simulink model "Bands7"  (R2018a)
settings: Solver=VariableStepAuto  StartTime=0.0  StopTime=0.01  RelTol=1e-3
undefined symbols (not defined in the file): fdesignblkfcn, G1, G2, G3, G4, G5, G6, G7, gcbh, get, T
libraries: dspsrcs4 x1, dspxfrm3 x1, dspobslib x1
(part 1 of 2)
settings Model: Creator=Daniel  LastModifiedBy=Daniel

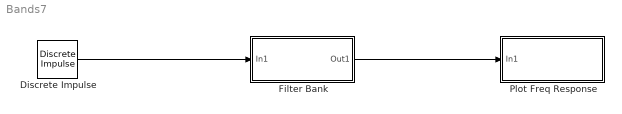
== system Bands7 ==
  Discrete Impulse : dspsrcs4/Discrete  Impulse  Delay=0  SampleTime=T  FrameSample=128  OutputFrames=off  dataType=double  isSigned=on  wordLen=16  udDataType=sfix(16)  fracBitsMode=Best precision  numFracBits=15  OutDataTypeStr=double  LastOutDataTypeStr=double
  "Filter Bank " : Subsystem
  Plot Freq Response : Subsystem
  wires:
  Discrete Impulse/1 -> "Filter Bank "/1(In1)
  "Filter Bank "/1(Out1) -> Plot Freq Response/1(In1)

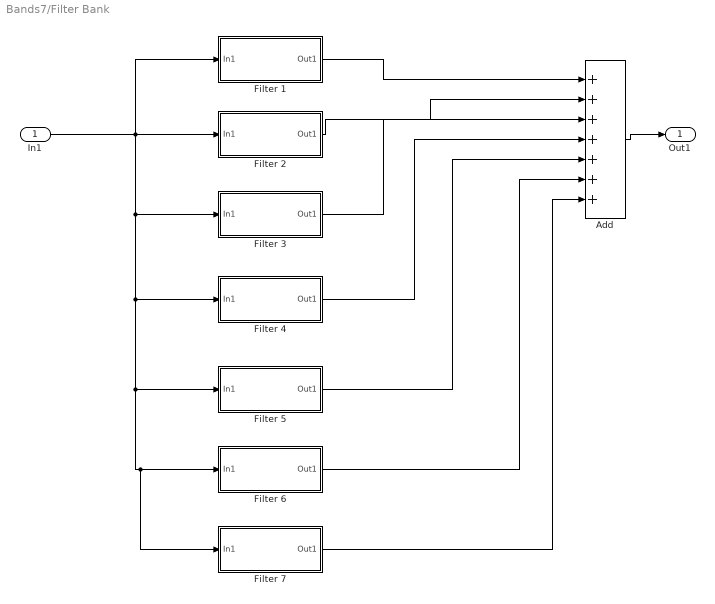
== system Bands7/Filter Bank  ==
  In1 : Inport
  Add : Sum  Inputs=+++++++
  Filter 1 : Subsystem
  Filter 2 : Subsystem
  Filter 3 : Subsystem
  Filter 4 : Subsystem
  Filter 5 : Subsystem
  Filter 6 : Subsystem
  Filter 7 : Subsystem
  Out1 : Outport
  wires:
  In1/1 -> Filter 3/1(In1), Filter 7/1(In1), Filter 6/1(In1), Filter 5/1(In1), Filter 4/1(In1), Filter 1/1(In1), Filter 2/1(In1)
  Add/1 -> Out1/1
  Filter 1/1(Out1) -> Add/1
  Filter 2/1(Out1) -> Add/2
  Filter 3/1(Out1) -> Add/3
  Filter 4/1(Out1) -> Add/4
  Filter 5/1(Out1) -> Add/5
  Filter 6/1(Out1) -> Add/6
  Filter 7/1(Out1) -> Add/7

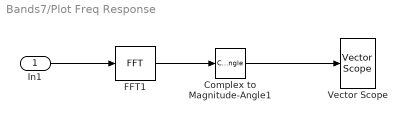
== system Bands7/Plot Freq Response ==
  In1 : Inport
  Complex to Magnitude-Angle1 : ComplexToMagnitudeAngle  Output=Magnitude
  FFT1 : dspxfrm3/FFT  FFTImplementation=Auto  CompMethod=Table lookup  TableOpt=NEW  TableOptActive=Speed  BitRevOrder=off  Normalize=off  InheritFFTLength=on  FFTLength=64  WrapInput=on  roundingMode=Floor  overflowMode=off  firstCoeffDataTypeStr=Inherit: Same word length as input  firstCoeffLastDataTypeStr=Inherit: Same word length as input  outputMin=[]  outputMax=[]
  Vector Scope : dspobslib/Vector Scope  ScopeProperties=off  Domain=Frequency  HorizSpan=1  DisplayProperties=off  AxisGrid=on  Memory=off  FrameNumber=off  AxisLegend=off  AxisZoom=off  OpenScopeAtSimStart=on  OpenScopeImmediately=off  FigPos=get(0,'defaultfigureposition')  AxisProperties=on  XUnits=Hertz  XRange=[0...Fs/2]  InheritXIncr=on  XIncr=1  XLabel=Samples  XLimit=Auto  XMin=0  XMax=1  XStart=0  YUnits=dB  YLabel=|Magnitude (dB)|  LineProperties=off  XAxisParamsVer=6.9
      settings: SourceProductName=DSP System Toolbox  SourceProductBaseCode=DS  YMin=0.0723692553519949  YMax=69.3188381671759
  wires:
  In1/1 -> FFT1/1
  FFT1/1 -> Complex to Magnitude-Angle1/1
  Complex to Magnitude-Angle1/1 -> Vector Scope/1

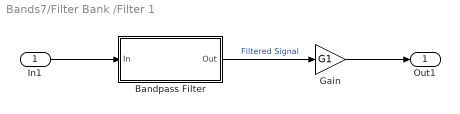
== system Bands7/Filter Bank /Filter 1 ==
  In1 : Inport
  Bandpass Filter : Subsystem  DialogController=fdesignblkfcn  InitFcn=fdesignblkfcn(gcbh, {'InitFcn'});  mask(Bandpass Filter){}
      mask help: Design a bandpass filter
      settings: CopyFcn=fdesignblkfcn(gcbh, {'CopyFcn'});
      mask Help: helpview(mapfilelocation('dsp'), 'dspbandpassfilter');
      mask Display: disp('Bandpass');
  Gain : Gain  Gain=G1
  Out1 : Outport
  wires:
  Bandpass Filter/1(Out) -> Gain/1  "Filtered Signal"
  In1/1 -> Bandpass Filter/1(In)
  Gain/1 -> Out1/1

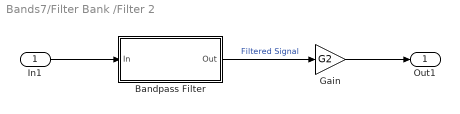
== system Bands7/Filter Bank /Filter 2 ==
  In1 : Inport
  Bandpass Filter : Subsystem  DialogController=fdesignblkfcn  InitFcn=fdesignblkfcn(gcbh, {'InitFcn'});  mask(Bandpass Filter){}
      mask help: Design a bandpass filter
      settings: CopyFcn=fdesignblkfcn(gcbh, {'CopyFcn'});
      mask Help: helpview(mapfilelocation('dsp'), 'dspbandpassfilter');
      mask Display: disp('Bandpass');
  Gain : Gain  Gain=G2
  Out1 : Outport
  wires:
  Bandpass Filter/1(Out) -> Gain/1  "Filtered Signal"
  In1/1 -> Bandpass Filter/1(In)
  Gain/1 -> Out1/1

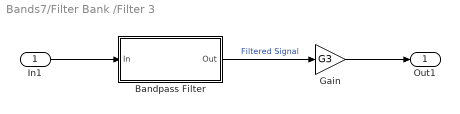
== system Bands7/Filter Bank /Filter 3 ==
  In1 : Inport
  Bandpass Filter : Subsystem  DialogController=fdesignblkfcn  InitFcn=fdesignblkfcn(gcbh, {'InitFcn'});  mask(Bandpass Filter){}
      mask help: Design a bandpass filter
      settings: CopyFcn=fdesignblkfcn(gcbh, {'CopyFcn'});
      mask Help: helpview(mapfilelocation('dsp'), 'dspbandpassfilter');
      mask Display: disp('Bandpass');
  Gain : Gain  Gain=G3
  Out1 : Outport
  wires:
  Bandpass Filter/1(Out) -> Gain/1  "Filtered Signal"
  In1/1 -> Bandpass Filter/1(In)
  Gain/1 -> Out1/1

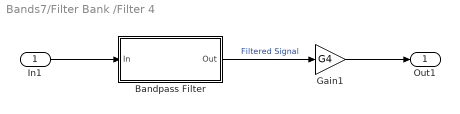
== system Bands7/Filter Bank /Filter 4 ==
  In1 : Inport
  Bandpass Filter : Subsystem  DialogController=fdesignblkfcn  InitFcn=fdesignblkfcn(gcbh, {'InitFcn'});  mask(Bandpass Filter){}
      mask help: Design a bandpass filter
      settings: CopyFcn=fdesignblkfcn(gcbh, {'CopyFcn'});
      mask Help: helpview(mapfilelocation('dsp'), 'dspbandpassfilter');
      mask Display: disp('Bandpass');
  Gain1 : Gain  Gain=G4
  Out1 : Outport
  wires:
  Bandpass Filter/1(Out) -> Gain1/1  "Filtered Signal"
  In1/1 -> Bandpass Filter/1(In)
  Gain1/1 -> Out1/1

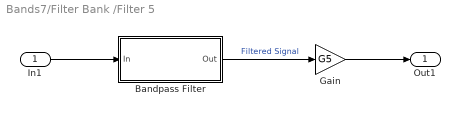
== system Bands7/Filter Bank /Filter 5 ==
  In1 : Inport
  Bandpass Filter : Subsystem  DialogController=fdesignblkfcn  InitFcn=fdesignblkfcn(gcbh, {'InitFcn'});  mask(Bandpass Filter){}
      mask help: Design a bandpass filter
      settings: CopyFcn=fdesignblkfcn(gcbh, {'CopyFcn'});
      mask Help: helpview(mapfilelocation('dsp'), 'dspbandpassfilter');
      mask Display: disp('Bandpass');
  Gain : Gain  Gain=G5
  Out1 : Outport
  wires:
  Bandpass Filter/1(Out) -> Gain/1  "Filtered Signal"
  In1/1 -> Bandpass Filter/1(In)
  Gain/1 -> Out1/1

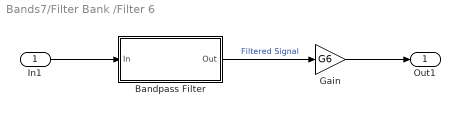
== system Bands7/Filter Bank /Filter 6 ==
  In1 : Inport
  Bandpass Filter : Subsystem  DialogController=fdesignblkfcn  InitFcn=fdesignblkfcn(gcbh, {'InitFcn'});  mask(Bandpass Filter){}
      mask help: Design a bandpass filter
      settings: CopyFcn=fdesignblkfcn(gcbh, {'CopyFcn'});
      mask Help: helpview(mapfilelocation('dsp'), 'dspbandpassfilter');
      mask Display: disp('Bandpass');
  Gain : Gain  Gain=G6
  Out1 : Outport
  wires:
  Bandpass Filter/1(Out) -> Gain/1  "Filtered Signal"
  In1/1 -> Bandpass Filter/1(In)
  Gain/1 -> Out1/1

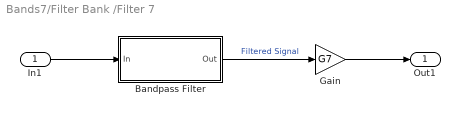
== system Bands7/Filter Bank /Filter 7 ==
  In1 : Inport
  Bandpass Filter : Subsystem  DialogController=fdesignblkfcn  InitFcn=fdesignblkfcn(gcbh, {'InitFcn'});  mask(Bandpass Filter){}
      mask help: Design a bandpass filter
      settings: CopyFcn=fdesignblkfcn(gcbh, {'CopyFcn'});
      mask Help: helpview(mapfilelocation('dsp'), 'dspbandpassfilter');
      mask Display: disp('Bandpass');
  Gain : Gain  Gain=G7
  Out1 : Outport
  wires:
  Bandpass Filter/1(Out) -> Gain/1  "Filtered Signal"
  In1/1 -> Bandpass Filter/1(In)
  Gain/1 -> Out1/1

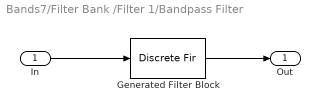
== system Bands7/Filter Bank /Filter 1/Bandpass Filter ==
  In : Inport
  Generated Filter Block : DiscreteFir  Tag=BlockMethodSubSystem  Coefficients=[-8.1048977494951512e-06 -2.43516407722459775e-05 -5.78898007116267508e-05 -0.000117381146531137762 -0.000213232473889349576 -0.000356076050289026833 -0.000555081789829506831 -0.00081583735031767312 -0.00113805071208230375 -0.00151348835005841054 -0.0019245122816521818 -0.00234372862013557896 -0.00273505385055416777 -0.00305643325395723621 -0.00326410312191345673 -0.00331809433073924952 -0.00318831155051930949 -0.00286032569228984474 -0.00233988805033344361 -0.00165522556282817271 -0.000856379714714089989 -1.12253504369335052e-05 0.0008016649044607358 0.00150261138447176437 0.00202165691315135112 0.00230906154108128248 0.00234373906668669313 0.00213807047179556632 0.00173797315251472077 0.00121778513617832955 0.000670368640632062118 0.000193678608696191891 -0.000124232758403682166 -0.000219389312514426239 -6.2800253190992486e-05 0.000333930798955978656 0.000919558050247468845 0.0016108905659800196 0.00230624165522150043 0.00290254563408762082 0.00331328238433551379 0.00348405103875359468 0.00340289253006853185 0.00310327189997440002 0.0026588758640486666 0.00217085993642671419 0.00174961399581836604 0.00149423753421569949 0.0014734923626712141 0.0017118865161618224 0.00218373121428606411 0.00281660799222071103 0.00350394143517449887 0.00412459426187716284 0.00456595741223267664 0.00474617167452667365 0.00463110659438667732 0.00424255899790257872 0.00365571589825402794 0.00298595951627125258 0.00236720799803940294 0.00192575934679139267 0.00175467286975830757 0.00189382960017879932 0.00231989661996557378 0.00294861641103723532 0.00364947042630501444 0.00427027501463488838 0.00466715793541905982 0.00473407565472849616 0.0044258715981516086 0.00376991996132528158 0.00286350355716879709 0.00185684497194729009 0.000924631555703508035 0.000231343012464668279 -0.000102804443773682285 -2.83101758387189872e-05 0.000420509863369374754 0.00112904228502097299 0.00192252842507701044 0.00259944974775010379 0.00297187963252515614 0.0029048204073523114 0.0023463930350089532 0.00134225826297456642 3.05927411666050058e-05 -0.00138222160874104097 -0.00266105531319380277 -0.00358918725245281275 -0.00401378022051056531 -0.00388021723480723706 -0.00324770117644405075 -0.00228204090876770686 -0.00122606673050510264 -0.000352762432933393299 8.99955315268397623e-05 -6.79491376219867193e-05 -0.000880072411975865395 -0.0022665599462196955 -0.00402452694290426124 -0.00586421077243191261 -0.0074648647805938273 -0.00853971159620926616 -0.00889693461758592034 -0.00848388928811058367 -0.00740457599388478702 -0.00590547459695627518 -0.00433115082853492532 -0.00305736929204881991 -0.00241447466112191221 -0.00261643906950001634 -0.00371055142781143502 -0.00555919163722859693 -0.0078590585292884884 -0.0101957446328822202 -0.0121241352104876302 -0.0132592952167562596 -0.0133595626610746396 -0.012384249427707052 -0.0105126909545392357 -0.00811868355247184759 -0.00570324242967302185 -0.00379736596180029222 -0.00285329105937439775 -0.00314608298568710542 -0.0047064482708399696 -0.00730036988827754453 -0.0104623892904168285 -0.0135787170491745452 -0.0160059089011951108 -0.0172027442990908309 -0.016848957113156527 -0.0149256340872515048 -0.0117384512920174645 -0.00787546895299421658 -0.00410403982477567774 -0.00122405220661133654 9.53435061134842233e-05 -0.000536674442832162112 -0.00313176427222673116 -0.0072919920286464799 -0.012260847254272041 -0.0170511501597739555 -0.0206296307164946027 -0.0221253070082664156 -0.0210218015234540333 -0.0172941123419765065 -0.0114584490963853067 -0.00451843994500049015 0.00219013994842459387 0.00723433696658829124 0.00936018226490840238 0.00776104937437556777 0.00228724823726593647 -0.00644671150652667297 -0.0170848980538309235 -0.0276886719972963616 -0.0360131619591159691 -0.0398612762771325957 -0.0374590614742793884 -0.0277894625492688258 -0.0108255451507139177 0.0123813099429946737 0.0397800429696240007 0.06855998131913911 0.0955198414511258531 0.117510882093258384 0.131885891803249833 0.136883388848354826 0.131885891803249833 ...(+3934 chars)]  InputProcessing=Columns as channels (frame based)
  Out : Outport
  wires:
  In/1 -> Generated Filter Block/1
  Generated Filter Block/1 -> Out/1

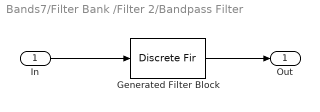
== system Bands7/Filter Bank /Filter 2/Bandpass Filter ==
  In : Inport
  Generated Filter Block : DiscreteFir  Tag=BlockMethodSubSystem  Coefficients=[-7.73471734753273964e-07 -1.8614193645339823e-06 -2.62993162904760566e-06 -1.38021866691025473e-06 3.65073568146082551e-06 1.26830114246925421e-05 2.26008331066257635e-05 2.64485043777322594e-05 1.56579925189179127e-05 -1.47529809869690204e-05 -5.99073741797206968e-05 -0.00010162016412352947 -0.000111954620278289011 -6.54017912315627107e-05 4.37217750731923579e-05 0.000187259521521445662 0.000303123154478809388 0.000315614026508990401 0.000172735184387801636 -0.000114720458756506374 -0.000454506862919527041 -0.000693008138340458829 -0.000676238169246097618 -0.000331156445314687996 0.00027127113267321314 0.000911064704961533542 0.00129111610742313585 0.00116770812102993862 0.000485094867947560599 -0.000555378019587216432 -0.00154155945159936735 -0.00201147287293983613 -0.00166806072656943967 -0.000547970627871920851 0.000947953034613348397 0.00219765265844689122 0.00262561153088946208 0.00197702589601981768 0.00046347106397167119 -0.0013033128878809305 -0.0025731690125243979 -0.00279856274465781424 -0.00189129915709874519 -0.000265471175711874772 0.0013597362660187043 0.00230244773239643517 0.00223483165715191367 0.00131513390080374975 7.21196485443082689e-05 -0.000890313403955640312 -0.00120594809653298916 -0.000908083414158724635 -0.000359026047450475706 2.01652239201366476e-06 -6.06896450353475037e-05 -0.000438008622209515015 -0.000756999443601519511 -0.000634289564126079087 5.37272742755294757e-05 0.00105308481203098491 0.0018477662527308287 0.00194950946767009936 0.00119401919953045265 -0.000135275965059666967 -0.00143809114668074075 -0.00211545272769665671 -0.00189412303621665917 -0.000968033856053282385 0.000127268354476420834 0.000833143201815613214 0.000889067797436123865 0.000463485885633809099 1.62133658949485818e-05 -2.08312245084271969e-05 0.0004564526785770583 0.00113638514213114405 0.00147887452130567726 0.00106848415402102962 -8.63462075097289397e-05 -0.00150316426650815927 -0.00247147468451690408 -0.00245793435977394821 -0.00142816915008616655 0.000115777121066530417 0.00141491548718761804 0.00188769619218162664 0.00145730664169443328 0.000570190116282471866 -0.000107874128074784181 -0.000129994351181496266 0.000436398302182251449 0.00105022731104654197 0.00105750884520188111 0.000149467739976468606 -0.00137705982557975249 -0.00273879535431928271 -0.0031121469816649287 -0.00214200832846823345 -0.000195550008219099456 0.00181112556972267704 0.00292499111706424637 0.00270288158454577362 0.00145701836667523925 4.16529467969392237e-05 -0.00069291216633277585 -0.000439446050715910658 0.000378032204521721595 0.00089654553086399491 0.000411355381501451165 -0.00110166242188334228 -0.0028866524891001384 -0.00382264432183298869 -0.00311623423801291044 -0.000843961692955167157 0.00201082560586479274 0.00407891301761270642 0.0043862128156380081 0.0029206060376847638 0.000627031331999448882 -0.00117936913938976188 -0.00162583180675710134 -0.000811129919751422653 0.000291694107547546988 0.00051066749145850499 -0.000694977610886266862 -0.00279056755466510842 -0.00442202890874845989 -0.00424692539912467377 -0.00183508623452647711 0.00194027283725385939 0.00530562963087596266 0.0065778415192755315 0.00515257484054923182 0.00187490281279850592 -0.001459459139687054 -0.00318525703197738335 -0.00276697676880172756 -0.00108355078289568271 0.000197768267945831207 -0.000224166678682294535 -0.00234013625154704495 -0.00472974385212686105 -0.00541803165005975539 -0.00318506098530876554 0.00150020811203707282 0.00655717514496674189 0.00940482388495060204 0.00846947630003617828 0.00416410665370636583 -0.00129825722025233214 -0.0051876582597605702 -0.00587240746293875467 -0.00376271073882080949 -0.000969408151197849758 0.000136442863038702128 -0.00143741987730687114 -0.00453523549555567666 -0.00650819254758591096 -0.00494827345320256531 0.000570790915992142544 0.00789278361387562612 0.013304776375525719 0.0136601593629206586 0.0083303881646475432 -0.000256397193257099456 -0.0079113279263046711 -0.0111004739583284821 ...(+5599 chars)]  InputProcessing=Columns as channels (frame based)
  Out : Outport
  wires:
  In/1 -> Generated Filter Block/1
  Generated Filter Block/1 -> Out/1

== system Bands7/Filter Bank /Filter 3/Bandpass Filter ==
  In : Inport
  Generated Filter Block : DiscreteFir  Tag=BlockMethodSubSystem  Coefficients=[-3.81639019890488076e-07 -9.13075038321544792e-07 -4.97880196082379438e-07 2.06238701435018126e-06 5.46179664005167287e-06 4.6731738347551529e-06 -4.79878573038164194e-06 -1.84562085027132781e-05 -2.01318863397847709e-05 4.7191379220310035e-06 4.57920595081008104e-05 6.12519464344169487e-05 1.06295026920179042e-05 -8.95118475435135519e-05 -0.000147657434599799385 -6.6054598037299276e-05 0.000140309387326405135 0.000297717561769824583 0.000198480855773592246 -0.000169494890882181137 -0.000515968607621079215 -0.000448069680157296962 0.000126570314026548284 0.000778521781696229023 0.000839728258821987369 5.14976313717255838e-05 -0.00102425982458233017 -0.00135929406545597532 -0.000416301862037827891 0.0011615028617581089 0.00193533555272718395 0.000974211777731036799 -0.00109567914993971408 -0.00244039151798019788 -0.00165663834110643237 0.000773667466540558916 0.00272122921992379264 0.00231328878083459765 -0.000228074701410981582 -0.00265518191876694789 -0.00274301747822173082 -0.000403117070534888947 0.0022132324403602451 0.00276172396366477406 0.000902426256722356382 -0.00149884502487769339 -0.00228563417393815808 -0.0010474521810633138 0.00073380583301770367 0.00139196569097000994 0.000711165564572970119 -0.000182268577851521458 -0.00031906999345782946 5.68367358107932117e-05 3.58070212730051855e-05 -0.000609893760065100183 -0.00101563346160873664 -0.000310290102283927705 0.00111821534859725619 0.00180871363540675736 0.00081203006338596373 -0.00110505046997391287 -0.00211046816267804064 -0.00120605312961525441 0.000704674010703898023 0.00178073524404852085 0.00116996368493228449 -0.000232081724521865981 -0.000947611619791236459 -0.000565854946607804478 2.65310617915142413e-05 -3.6442434989779732e-05 -0.000460251524579809396 -0.000264065802570286068 0.00075910954405309847 0.00151738182892546336 0.000839670539656595062 -0.000958605678978728996 -0.0021458076723046139 -0.00139605748720050523 0.000668164789717689959 0.00205122669056761152 0.0015033277827929516 -0.000204990095625071312 -0.00127304445377434002 -0.000906509601534579747 -7.6165738077278694e-06 0.000183869869175824573 -0.000294041905629426363 -0.000300612092719415277 0.000697930721759493894 0.0016441951804494761 0.00105204506351403186 -0.000993251690669912438 -0.00254270358623776612 -0.00181717541641454225 0.000686612764101606171 0.00255751886523889914 0.0020298731354438126 -0.000148898502636345722 -0.00167865079088852574 -0.00132075223960171663 -7.73089621244891682e-05 0.000350928645032154397 -0.000218418352662667361 -0.000375483600942958179 0.000756300285359090422 0.00200981087933193485 0.0014211790316228884 -0.00113098995618473772 -0.00325145117868610696 -0.00249429074801465166 0.000734470371698941571 0.00334450569590704705 0.00282876057830729272 -4.94273856107960201e-05 -0.00224822803040351663 -0.00191057412044807486 -0.000200292313597152748 0.000539949799661205597 -0.000152846889558606023 -0.000479795795959799248 0.00088812835498835042 0.00258700167066069995 0.00196927428465709306 -0.00134772033564384665 -0.00430091688188779121 -0.00349066462516963837 0.000790213754854437967 0.00447143521985536932 0.00398784282104593969 0.000122815378689030541 -0.00303401829798591489 -0.00274829268862077352 -0.000401606059962189067 0.000770293313358233912 -8.50480490386363951e-05 -0.000624508619439108695 0.00110558707308841043 0.00344669130738582729 0.00277425786200690295 -0.00166068793366865551 -0.00582978802456672173 -0.00495493927979833923 0.000845197899938326665 0.00609372710657809027 0.00568623301322510911 0.000409503883480374442 -0.00414640980672515477 -0.00396578043505057317 -0.000721019843669409551 0.00107012962122787813 -1.3343948743235347e-05 -0.000841266561696989395 0.00144982006639912957 0.00476029418198006728 0.0040064648822888153 -0.00212066545884323238 -0.00815093589214566962 -0.00720903479741472758 0.000891405811849098752 0.00855984092420954482 0.0083167131843229769 0.00089648950199610407 -0.00583408073857200667 -0.00585601954256646101 -0.00124662048010526385 ...(+6266 chars)]  InputProcessing=Columns as channels (frame based)
  Out : Outport
  wires:
  In/1 -> Generated Filter Block/1
  Generated Filter Block/1 -> Out/1

== system Bands7/Filter Bank /Filter 4/Bandpass Filter ==
  In : Inport
  Generated Filter Block : DiscreteFir  Tag=BlockMethodSubSystem  Coefficients=[-7.38876505953358568e-08 3.13348726053644364e-08 3.93571493384327713e-07 2.38131173681242125e-07 -9.51531478599497375e-07 -1.25903148753861206e-06 1.43099993629581749e-06 3.64770495032386579e-06 -8.00265292323240663e-07 -7.63757899433189141e-06 -2.71265899838620468e-06 1.24130486409139518e-05 1.12379095838631487e-05 -1.54543243618824984e-05 -2.63199333463828875e-05 1.23031998748595195e-05 4.75937622428491852e-05 2.96996576262737109e-06 -7.14149717603653497e-05 -3.64955516820133135e-05 8.97959556523460656e-05 9.25550789741004634e-05 -8.99528018903434561e-05 -0.000170747147757154748 5.48929924101161101e-05 0.000262365873845357049 3.4105818749502325e-05 -0.000346446866615849648 -0.000191880407191225629 0.000387150870603270795 0.000419815637651545692 -0.000335746779465051362 -0.000693564612294760496 0.00014110793640943574 0.000952852041716606532 0.000229377955587480248 -0.00110150845829050251 -0.000762085381563493819 0.00102599869677799335 0.0013736628496103661 -0.000634945306791181042 -0.00190798228316189184 -8.9318165229259556e-05 0.00216733510138123744 0.00104872503556306652 -0.00197893501222640373 -0.00202428618737933745 0.00127773201491330557 0.0027266298034902374 -0.000168769303023740929 -0.00289752451963061833 -0.00107080353716598763 0.00242734529822534201 0.00207058795815893894 -0.00143281843841261912 -0.00250913077694213523 0.000244458632121062657 0.00226217756182780713 0.000711026651859420736 -0.00148182110409991632 -0.00109413570459319714 0.00055215413674032036 0.000818038354689593766 7.61589643096634636e-05 -0.000106192442645053128 -0.000102689796674200628 -0.000603483047154900571 -0.000464143133500814981 0.000874820819663964851 0.00129956323798973046 -0.000504558762396600607 -0.00192557866238567241 -0.000358690426553892789 0.00196901118813915151 0.00128468642491254325 -0.0013754911207042894 -0.00179597880585333105 0.00045233631089153112 0.0016423773744013929 0.000297310402984651628 -0.000956288065582377327 -0.000465005500254926836 0.000187881389338045242 -1.43673494172366505e-05 0.000155142334820137828 0.000810065778978096116 0.000183687101971264798 -0.00138392605224316395 -0.00104048755672205115 0.00131764676127290822 0.00191612609235892735 -0.000581878271795050199 -0.00227774102630577116 -0.000427249728666408558 0.0018981951052163173 0.00112222904075565903 -0.0010178168134932161 -0.00109522718860560384 0.000212330798290565943 0.00039396282471938944 -3.38895491342412801e-05 0.000484211421277762311 0.000645583693702266341 -0.000894943692433727042 -0.00169004715443951269 0.000466246114925255098 0.00249528932426618501 0.000636057552963867714 -0.00250410006410799711 -0.0017847892764979278 0.0016555639567511517 0.00228285707385448861 -0.000459043601357273672 -0.00182906527934257115 -0.000311576931333359703 0.000749305424909547024 0.000124640860258760927 0.000180787401401104916 0.000930135604997572234 -0.000231943420378034383 -0.00215746665283858509 -0.000777344337328971088 0.00268656350559977981 0.00231571499737845583 -0.00205367837768387221 -0.00344892762010874741 0.000550455980979265742 0.00344968245151054936 0.000918901208595547373 -0.00231258286367762647 -0.00141226665284331469 0.000813078532997305752 0.000595282607983128398 -3.36357060198599312e-05 0.000980567071294485186 0.000640839659295775344 -0.00218853836540057901 -0.00239175043071141943 0.00205906301877590908 0.00422866662391428293 -0.000462526028422469886 -0.00494459852101824127 -0.00173346156163693937 0.00400595607797592755 0.0031840296926663892 -0.0019761590483461911 -0.00296003174910024333 0.000214000771727097127 0.00122637113895656216 4.31023028709232077e-06 0.000782266443731995153 0.00162124037103426465 -0.0015301075610755588 -0.00412376323036092035 0.000222572128645609827 0.00583420126119994255 0.00257829287745940531 -0.00548189741952038491 -0.00522897018100930769 0.00311218985548222934 0.00605532990416025787 -0.000167600306790639559 -0.00451570281688404383 -0.00139633517420677581 0.00167719031551201068 0.000430093668416671449 0.000386432251526694034 ...(+6930 chars)]  InputProcessing=Columns as channels (frame based)
  Out : Outport
  wires:
  In/1 -> Generated Filter Block/1
  Generated Filter Block/1 -> Out/1
